simulink model "SingleIntegrator"  (R2015b)
settings: Solver=VariableStepAuto  StartTime=0.0  StopTime=10.0  RelTol=1e-3
settings Model: Creator=Wolfgang  LastModifiedBy=Wolfgang

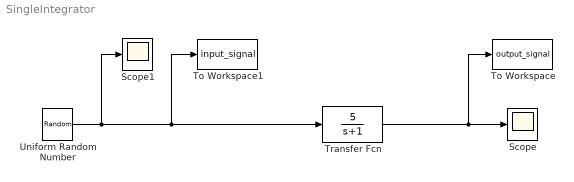
== system SingleIntegrator ==
  Scope : Scope
  Scope1 : Scope
  To Workspace : ToWorkspace  VariableName=output_signal  SampleTime=-1
      settings: Save2DSignal=2-D array (concatenate along first dimension)
  To Workspace1 : ToWorkspace  VariableName=input_signal  SampleTime=-1
  Transfer Fcn : TransferFcn  Numerator=[5]  Denominator=[1 1]
  Uniform Random Number : UniformRandomNumber  SampleTime=0.001
  wires:
  Uniform Random Number/1 -> Transfer Fcn/1, To Workspace1/1, Scope1/1
  Transfer Fcn/1 -> To Workspace/1, Scope/1
